simulink model "Simulation"  (R2019b)
settings: Solver=VariableStepAuto  StartTime=0.0  StopTime=tmax  RelTol=1e-3
values from neighbouring files (symbols this model uses):
  BPden = [1 alpha]    [RunSimulation.m]    (also in RunTest.m)
  BPnum = [0.3 alpha]    [RunSimulation.m]    (also in RunTest.m)
  c = 250    [RunSimulation.m]    (also in RunTest.m)
  efficiency = 0.95    [RunSimulation.m]
  Fb = -1*m    (= -90000)    [RunSimulation.m]
  l = 18    [RunSimulation.m]    (also in RunTest.m)
  m = 90000    [RunSimulation.m]
  p0 = 0    [RunSimulation.m]    (also in RunTest.m)
  Pres = 0/1000*[5.7/771 0 1.6]    [RunSimulation.m]    (also in RunTest.m)
  RBD = 5    [RunSimulation.m]    (also in RunTest.m)
  tl = .1    (= 0.1)    [RunSimulation.m]    (also in RunTest.m)
  trackgradient = 0    [RunSimulation.m]    (also in RunTest.m)
  trainpower = m    (= 90000)    [RunSimulation.m]
  v0 = 100/3.6    (= 27.7777777778)    [RunSimulation.m]
  VBD = 3.5    [RunSimulation.m]    (also in RunTest.m)
libraries: simulink x11
(part 1 of 5)
settings Model: Creator=raphael  LastModifiedBy=Westfechtel
settings DataIOCC: ReturnWorkspaceOutputs=off
settings DebuggingCC: ArithmeticOperatorsInVariantConditions=warning
settings SFSimCC: CustomCodeUndefinedFunction=UseInterfaceOnly

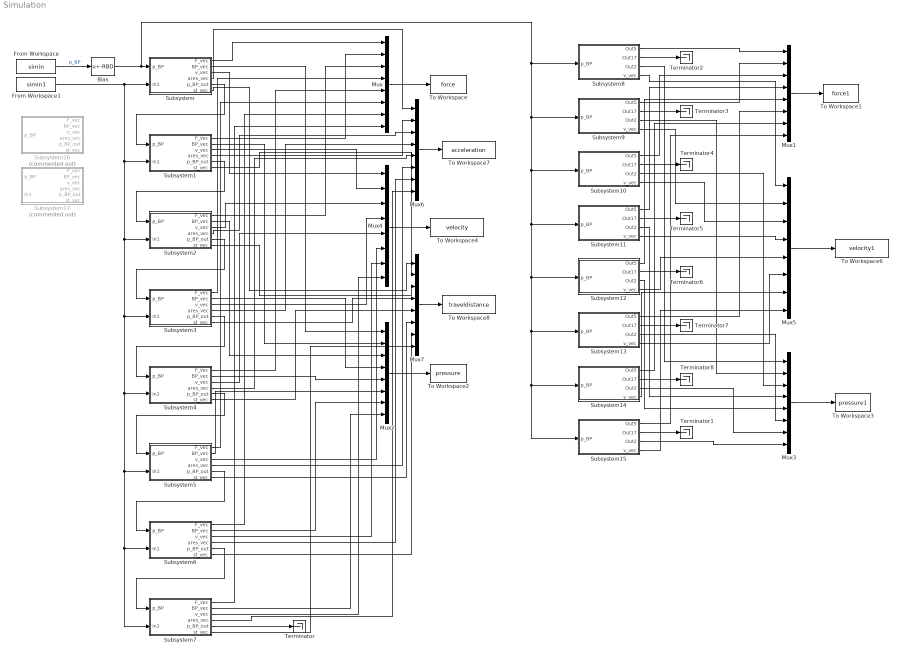
== system Simulation ==
  Bias : Bias  Bias=-RBD
  From Workspace : FromWorkspace  VariableName=simin  SampleTime=0
  From Workspace1 : FromWorkspace  VariableName=simin1  SampleTime=0
  Mux{,1..7} (8 alike) : Mux  Inputs=8
  Subsystem : Subsystem
  Subsystem1 : Subsystem
  Subsystem10 : Subsystem
  Subsystem11 : Subsystem
  Subsystem12 : Subsystem
  Subsystem13 : Subsystem
  Subsystem14 : Subsystem
  Subsystem15 : Subsystem
  Subsystem16 : Subsystem  Commented=on
  Subsystem17 : Subsystem  Commented=on
  Subsystem2 : Subsystem
  Subsystem3 : Subsystem
  Subsystem4 : Subsystem
  Subsystem5 : Subsystem
  Subsystem6 : Subsystem
  Subsystem7 : Subsystem
  Subsystem8 : Subsystem
  Subsystem9 : Subsystem
  Terminator{,1..8} (9 alike) : Terminator
  To Workspace : ToWorkspace  VariableName=force  SaveFormat=Timeseries  SampleTime=-1
  To Workspace1 : ToWorkspace  VariableName=force1  SaveFormat=Timeseries  SampleTime=-1
  To Workspace2 : ToWorkspace  VariableName=pressure  SaveFormat=Timeseries  SampleTime=-1
  To Workspace3 : ToWorkspace  VariableName=pressure1  SaveFormat=Timeseries  SampleTime=-1
  To Workspace4 : ToWorkspace  VariableName=velocity  SaveFormat=Timeseries  SampleTime=-1
  To Workspace6 : ToWorkspace  VariableName=velocity1  SaveFormat=Timeseries  SampleTime=-1
  To Workspace7 : ToWorkspace  VariableName=acceleration  SaveFormat=Timeseries  SampleTime=-1
  To Workspace8 : ToWorkspace  VariableName=traveldistance  SaveFormat=Timeseries  SampleTime=-1
  wires:
  Mux/1 -> To Workspace/1
  Mux2/1 -> To Workspace2/1
  From Workspace/1 -> Bias/1  "p_BP"
  Bias/1 -> Subsystem15/1(p_BP), Subsystem14/1(p_BP), Subsystem13/1(p_BP), Subsystem12/1(p_BP), Subsystem11/1(p_BP), Subsystem10/1(p_BP), Subsystem9/1(p_BP), Subsystem8/1(p_BP), Subsystem/1(p_BP)
  Mux1/1 -> To Workspace1/1
  Mux3/1 -> To Workspace3/1
  Mux4/1 -> To Workspace4/1
  Mux5/1 -> To Workspace6/1
  Subsystem8/2(Out17) -> Terminator2/1
  Subsystem9/2(Out17) -> Terminator3/1
  Subsystem10/2(Out17) -> Terminator4/1
  Subsystem11/2(Out17) -> Terminator5/1
  Subsystem12/2(Out17) -> Terminator6/1
  Subsystem13/2(Out17) -> Terminator7/1
  Subsystem14/2(Out17) -> Terminator8/1
  Subsystem15/2(Out17) -> Terminator1/1
  Subsystem/1(F_vec) -> Mux/1
  Subsystem8/1(Out5) -> Mux1/1
  Subsystem9/1(Out5) -> Mux1/2
  Subsystem10/1(Out5) -> Mux1/3
  Subsystem11/1(Out5) -> Mux1/4
  Subsystem12/1(Out5) -> Mux1/5
  Subsystem13/1(Out5) -> Mux1/6
  Subsystem14/1(Out5) -> Mux1/7
  Subsystem15/1(Out5) -> Mux1/8
  Subsystem8/3(Out2) -> Mux3/1
  Subsystem9/3(Out2) -> Mux3/2
  Subsystem10/3(Out2) -> Mux3/3
  Subsystem11/3(Out2) -> Mux3/4
  Subsystem12/3(Out2) -> Mux3/5
  Subsystem13/3(Out2) -> Mux3/6
  Subsystem14/3(Out2) -> Mux3/7
  Subsystem15/3(Out2) -> Mux3/8
  Subsystem8/4("v_vec ") -> Mux5/1
  Subsystem9/4("v_vec ") -> Mux5/2
  Subsystem10/4("v_vec ") -> Mux5/3
  Subsystem11/4("v_vec ") -> Mux5/4
  Subsystem12/4("v_vec ") -> Mux5/5
  Subsystem13/4("v_vec ") -> Mux5/6
  Subsystem14/4("v_vec ") -> Mux5/7
  Subsystem15/4("v_vec ") -> Mux5/8
  Subsystem7/5(p_BP_out) -> Terminator/1
  Subsystem/5(p_BP_out) -> Subsystem1/1(p_BP)
  Subsystem1/5(p_BP_out) -> Subsystem2/1(p_BP)
  Subsystem2/5(p_BP_out) -> Subsystem3/1(p_BP)
  Subsystem3/5(p_BP_out) -> Subsystem4/1(p_BP)
  Subsystem4/5(p_BP_out) -> Subsystem5/1(p_BP)
  Subsystem5/5(p_BP_out) -> Subsystem6/1(p_BP)
  Subsystem6/5(p_BP_out) -> Subsystem7/1(p_BP)
  Subsystem/2(BP_vec) -> Mux2/1
  Subsystem1/2(BP_vec) -> Mux2/2
  Subsystem1/1(F_vec) -> Mux/2
  Subsystem2/1(F_vec) -> Mux/3
  Subsystem3/1(F_vec) -> Mux/4
  Subsystem4/1(F_vec) -> Mux/5
  Subsystem5/1(F_vec) -> Mux/6
  Subsystem6/1(F_vec) -> Mux/7
  Subsystem7/1(F_vec) -> Mux/8
  Subsystem2/2(BP_vec) -> Mux2/3
  Subsystem3/2(BP_vec) -> Mux2/4
  Subsystem4/2(BP_vec) -> Mux2/5
  Subsystem5/2(BP_vec) -> Mux2/6
  Subsystem6/2(BP_vec) -> Mux2/7
  Subsystem7/2(BP_vec) -> Mux2/8
  Subsystem/3(v_vec) -> Mux4/1
  Subsystem1/3(v_vec) -> Mux4/2
  Subsystem2/3(v_vec) -> Mux4/3
  Subsystem3/3(v_vec) -> Mux4/4
  Subsystem4/3(v_vec) -> Mux4/5
  Subsystem5/3(v_vec) -> Mux4/6
  Subsystem6/3(v_vec) -> Mux4/7
  Subsystem7/3(v_vec) -> Mux4/8
  Mux6/1 -> To Workspace7/1
  Mux7/1 -> To Workspace8/1
  Subsystem/4(ares_vec) -> Mux6/1
  Subsystem1/4(ares_vec) -> Mux6/2
  Subsystem2/4(ares_vec) -> Mux6/3
  Subsystem3/4(ares_vec) -> Mux6/4
  Subsystem4/4(ares_vec) -> Mux6/5
  Subsystem5/4(ares_vec) -> Mux6/6
  Subsystem6/4(ares_vec) -> Mux6/7
  Subsystem7/4(ares_vec) -> Mux6/8
  Subsystem/6(st_vec) -> Mux7/1
  Subsystem1/6(st_vec) -> Mux7/2
  Subsystem2/6(st_vec) -> Mux7/3
  Subsystem3/6(st_vec) -> Mux7/4
  Subsystem4/6(st_vec) -> Mux7/5
  Subsystem5/6(st_vec) -> Mux7/6
  Subsystem6/6(st_vec) -> Mux7/7
  Subsystem7/6(st_vec) -> Mux7/8
  From Workspace1/1 -> Subsystem/2(In1), Subsystem1/2(In1), Subsystem2/2(In1), Subsystem3/2(In1), Subsystem4/2(In1), Subsystem5/2(In1), Subsystem7/2(In1), Subsystem6/2(In1)

== system Simulation/Subsystem ==
  p_BP : Inport
  In1 : Inport  Port=2
  Mux{,1..4} (5 alike) : Mux  Inputs=5
  Wagon model : Subsystem
  Wagon model1 : Subsystem
  Wagon model2 : Subsystem
  Wagon model3 : Subsystem
  Wagon model4 : Subsystem
  F_vec : Outport  VectorParamsAs1DForOutWhenUnconnected=off
  BP_vec : Outport  Port=2  VectorParamsAs1DForOutWhenUnconnected=off
  v_vec : Outport  Port=3  VectorParamsAs1DForOutWhenUnconnected=off
  ares_vec : Outport  Port=4  VectorParamsAs1DForOutWhenUnconnected=off
  p_BP_out : Outport  Port=5  VectorParamsAs1DForOutWhenUnconnected=off
  st_vec : Outport  Port=6  VectorParamsAs1DForOutWhenUnconnected=off
  wires:
  Mux/1 -> F_vec/1  "F_vec"
  p_BP/1 -> Wagon model/1(p_BP)
  Mux1/1 -> BP_vec/1  "BP_vec"
  Mux2/1 -> v_vec/1  "v_vec"
  Mux3/1 -> ares_vec/1  "ares_vec"
  Wagon model4/2(p_BP_out) -> Mux1/5, p_BP_out/1  "p_BP_out"
  Wagon model/1(Fres) -> Mux/1
  Wagon model1/1(Fres) -> Mux/2
  Wagon model2/1(Fres) -> Mux/3
  Wagon model3/1(Fres) -> Mux/4
  Wagon model4/1(Fres) -> Mux/5
  Wagon model/2(p_BP_out) -> Wagon model1/1(p_BP), Mux1/1
  Wagon model1/2(p_BP_out) -> Wagon model2/1(p_BP), Mux1/2
  Wagon model2/2(p_BP_out) -> Wagon model3/1(p_BP), Mux1/3
  Wagon model3/2(p_BP_out) -> Wagon model4/1(p_BP), Mux1/4
  Wagon model/3("v ") -> Mux2/1
  Wagon model1/3("v ") -> Mux2/2
  Wagon model2/3("v ") -> Mux2/3
  Wagon model3/3("v ") -> Mux2/4
  Wagon model4/3("v ") -> Mux2/5
  Wagon model/4(ares) -> Mux3/1
  Wagon model1/4(ares) -> Mux3/2
  Wagon model2/4(ares) -> Mux3/3
  Wagon model3/4(ares) -> Mux3/4
  Wagon model4/4(ares) -> Mux3/5
  Mux4/1 -> st_vec/1  "st_vec"
  Wagon model/5(st) -> Mux4/1
  Wagon model1/5(st) -> Mux4/2
  Wagon model2/5(st) -> Mux4/3
  Wagon model3/5(st) -> Mux4/4
  Wagon model4/5(st) -> Mux4/5
  In1/1 -> Wagon model1/2(In1), Wagon model2/2(In1), Wagon model4/2(In1), Wagon model3/2(In1), Wagon model/2(In1)

== system Simulation/Subsystem1 ==
  p_BP : Inport
  In1 : Inport  Port=2
  Mux{,1..4} (5 alike) : Mux  Inputs=5
  Wagon model : Subsystem
  Wagon model1 : Subsystem
  Wagon model2 : Subsystem
  Wagon model3 : Subsystem
  Wagon model4 : Subsystem
  F_vec : Outport  VectorParamsAs1DForOutWhenUnconnected=off
  BP_vec : Outport  Port=2  VectorParamsAs1DForOutWhenUnconnected=off
  v_vec : Outport  Port=3  VectorParamsAs1DForOutWhenUnconnected=off
  ares_vec : Outport  Port=4  VectorParamsAs1DForOutWhenUnconnected=off
  p_BP_out : Outport  Port=5  VectorParamsAs1DForOutWhenUnconnected=off
  st_vec : Outport  Port=6  VectorParamsAs1DForOutWhenUnconnected=off
  wires:
  Mux/1 -> F_vec/1  "F_vec"
  p_BP/1 -> Wagon model/1(p_BP)
  Mux1/1 -> BP_vec/1  "BP_vec"
  Mux2/1 -> v_vec/1  "v_vec"
  Mux3/1 -> ares_vec/1  "ares_vec"
  Wagon model4/2(p_BP_out) -> Mux1/5, p_BP_out/1  "p_BP_out"
  Wagon model/1(Fres) -> Mux/1
  Wagon model1/1(Fres) -> Mux/2
  Wagon model2/1(Fres) -> Mux/3
  Wagon model3/1(Fres) -> Mux/4
  Wagon model4/1(Fres) -> Mux/5
  Wagon model/2(p_BP_out) -> Wagon model1/1(p_BP), Mux1/1
  Wagon model1/2(p_BP_out) -> Wagon model2/1(p_BP), Mux1/2
  Wagon model2/2(p_BP_out) -> Wagon model3/1(p_BP), Mux1/3
  Wagon model3/2(p_BP_out) -> Wagon model4/1(p_BP), Mux1/4
  Wagon model/3("v ") -> Mux2/1
  Wagon model1/3("v ") -> Mux2/2
  Wagon model2/3("v ") -> Mux2/3
  Wagon model3/3("v ") -> Mux2/4
  Wagon model4/3("v ") -> Mux2/5
  Wagon model/4(ares) -> Mux3/1
  Wagon model1/4(ares) -> Mux3/2
  Wagon model2/4(ares) -> Mux3/3
  Wagon model3/4(ares) -> Mux3/4
  Wagon model4/4(ares) -> Mux3/5
  Mux4/1 -> st_vec/1  "st_vec"
  Wagon model/5(st) -> Mux4/1
  Wagon model1/5(st) -> Mux4/2
  Wagon model2/5(st) -> Mux4/3
  Wagon model3/5(st) -> Mux4/4
  Wagon model4/5(st) -> Mux4/5
  In1/1 -> Wagon model1/2(In1), Wagon model2/2(In1), Wagon model4/2(In1), Wagon model3/2(In1), Wagon model/2(In1)

== system Simulation/Subsystem10 ==
  note: v_vec
  p_BP : Inport
  Mux : Mux  Inputs=5
  Mux1 : Mux  Inputs=5
  Mux2 : Mux  Inputs=5
  Wagon model : Subsystem
  Wagon model1 : Subsystem
  Wagon model2 : Subsystem
  Wagon model3 : Subsystem
  Wagon model4 : Subsystem
  Out5 : Outport  VectorParamsAs1DForOutWhenUnconnected=off
  Out17 : Outport  Port=2  VectorParamsAs1DForOutWhenUnconnected=off
  Out2 : Outport  Port=3  VectorParamsAs1DForOutWhenUnconnected=off
  "v_vec " : Outport  Port=4
  wires:
  Wagon model3/2(p_BP_out) -> Mux2/4, Wagon model4/1(p_BP)
  Mux/1 -> Out5/1  "F_vec"
  Wagon model1/2(p_BP_out) -> Mux2/2, Wagon model2/1(p_BP)
  Wagon model4/2(p_BP_out) -> Out17/1, Mux2/5  "p_BP_out"
  Wagon model4/1(Fres) -> Mux/5
  Wagon model2/2(p_BP_out) -> Mux2/3, Wagon model3/1(p_BP)
  Wagon model/2(p_BP_out) -> Mux2/1, Wagon model1/1(p_BP)
  Wagon model3/1(Fres) -> Mux/4
  Wagon model2/1(Fres) -> Mux/3
  Wagon model1/1(Fres) -> Mux/2
  Wagon model/1(Fres) -> Mux/1
  Mux2/1 -> Out2/1  "BP_vec"
  p_BP/1 -> Wagon model/1(p_BP)
  Wagon model/3("v ") -> Mux1/1
  Wagon model1/3("v ") -> Mux1/2
  Wagon model3/3("v ") -> Mux1/3
  Wagon model4/3("v ") -> Mux1/5
  Wagon model2/3("v ") -> Mux1/4
  Mux1/1 -> "v_vec "/1

== system Simulation/Subsystem11 ==
  note: v_vec
  p_BP : Inport
  Mux : Mux  Inputs=5
  Mux1 : Mux  Inputs=5
  Mux2 : Mux  Inputs=5
  Wagon model : Subsystem
  Wagon model1 : Subsystem
  Wagon model2 : Subsystem
  Wagon model3 : Subsystem
  Wagon model4 : Subsystem
  Out5 : Outport  VectorParamsAs1DForOutWhenUnconnected=off
  Out17 : Outport  Port=2  VectorParamsAs1DForOutWhenUnconnected=off
  Out2 : Outport  Port=3  VectorParamsAs1DForOutWhenUnconnected=off
  "v_vec " : Outport  Port=4
  wires:
  Wagon model3/2(p_BP_out) -> Mux2/4, Wagon model4/1(p_BP)
  Mux/1 -> Out5/1  "F_vec"
  Wagon model1/2(p_BP_out) -> Mux2/2, Wagon model2/1(p_BP)
  Wagon model4/2(p_BP_out) -> Out17/1, Mux2/5  "p_BP_out"
  Wagon model4/1(Fres) -> Mux/5
  Wagon model2/2(p_BP_out) -> Mux2/3, Wagon model3/1(p_BP)
  Wagon model/2(p_BP_out) -> Mux2/1, Wagon model1/1(p_BP)
  Wagon model3/1(Fres) -> Mux/4
  Wagon model2/1(Fres) -> Mux/3
  Wagon model1/1(Fres) -> Mux/2
  Wagon model/1(Fres) -> Mux/1
  Mux2/1 -> Out2/1  "BP_vec"
  p_BP/1 -> Wagon model/1(p_BP)
  Wagon model/3("v ") -> Mux1/1
  Wagon model1/3("v ") -> Mux1/2
  Wagon model3/3("v ") -> Mux1/3
  Wagon model4/3("v ") -> Mux1/5
  Wagon model2/3("v ") -> Mux1/4
  Mux1/1 -> "v_vec "/1

== system Simulation/Subsystem12 ==
  note: v_vec
  p_BP : Inport
  Mux : Mux  Inputs=5
  Mux1 : Mux  Inputs=5
  Mux2 : Mux  Inputs=5
  Wagon model : Subsystem
  Wagon model1 : Subsystem
  Wagon model2 : Subsystem
  Wagon model3 : Subsystem
  Wagon model4 : Subsystem
  Out5 : Outport  VectorParamsAs1DForOutWhenUnconnected=off
  Out17 : Outport  Port=2  VectorParamsAs1DForOutWhenUnconnected=off
  Out2 : Outport  Port=3  VectorParamsAs1DForOutWhenUnconnected=off
  "v_vec " : Outport  Port=4
  wires:
  Wagon model3/2(p_BP_out) -> Mux2/4, Wagon model4/1(p_BP)
  Mux/1 -> Out5/1  "F_vec"
  Wagon model1/2(p_BP_out) -> Mux2/2, Wagon model2/1(p_BP)
  Wagon model4/2(p_BP_out) -> Out17/1, Mux2/5  "p_BP_out"
  Wagon model4/1(Fres) -> Mux/5
  Wagon model2/2(p_BP_out) -> Mux2/3, Wagon model3/1(p_BP)
  Wagon model/2(p_BP_out) -> Mux2/1, Wagon model1/1(p_BP)
  Wagon model3/1(Fres) -> Mux/4
  Wagon model2/1(Fres) -> Mux/3
  Wagon model1/1(Fres) -> Mux/2
  Wagon model/1(Fres) -> Mux/1
  Mux2/1 -> Out2/1  "BP_vec"
  p_BP/1 -> Wagon model/1(p_BP)
  Wagon model/3("v ") -> Mux1/1
  Wagon model1/3("v ") -> Mux1/2
  Wagon model3/3("v ") -> Mux1/3
  Wagon model4/3("v ") -> Mux1/5
  Wagon model2/3("v ") -> Mux1/4
  Mux1/1 -> "v_vec "/1

== system Simulation/Subsystem13 ==
  note: v_vec
  p_BP : Inport
  Mux : Mux  Inputs=5
  Mux1 : Mux  Inputs=5
  Mux2 : Mux  Inputs=5
  Wagon model : Subsystem
  Wagon model1 : Subsystem
  Wagon model2 : Subsystem
  Wagon model3 : Subsystem
  Wagon model4 : Subsystem
  Out5 : Outport  VectorParamsAs1DForOutWhenUnconnected=off
  Out17 : Outport  Port=2  VectorParamsAs1DForOutWhenUnconnected=off
  Out2 : Outport  Port=3  VectorParamsAs1DForOutWhenUnconnected=off
  "v_vec " : Outport  Port=4
  wires:
  Wagon model3/2(p_BP_out) -> Mux2/4, Wagon model4/1(p_BP)
  Mux/1 -> Out5/1  "F_vec"
  Wagon model1/2(p_BP_out) -> Mux2/2, Wagon model2/1(p_BP)
  Wagon model4/2(p_BP_out) -> Out17/1, Mux2/5  "p_BP_out"
  Wagon model4/1(Fres) -> Mux/5
  Wagon model2/2(p_BP_out) -> Mux2/3, Wagon model3/1(p_BP)
  Wagon model/2(p_BP_out) -> Mux2/1, Wagon model1/1(p_BP)
  Wagon model3/1(Fres) -> Mux/4
  Wagon model2/1(Fres) -> Mux/3
  Wagon model1/1(Fres) -> Mux/2
  Wagon model/1(Fres) -> Mux/1
  Mux2/1 -> Out2/1  "BP_vec"
  p_BP/1 -> Wagon model/1(p_BP)
  Wagon model/3("v ") -> Mux1/1
  Wagon model1/3("v ") -> Mux1/2
  Wagon model3/3("v ") -> Mux1/3
  Wagon model4/3("v ") -> Mux1/5
  Wagon model2/3("v ") -> Mux1/4
  Mux1/1 -> "v_vec "/1

== system Simulation/Subsystem14 ==
  note: v_vec
  p_BP : Inport
  Mux : Mux  Inputs=5
  Mux1 : Mux  Inputs=5
  Mux2 : Mux  Inputs=5
  Wagon model : Subsystem
  Wagon model1 : Subsystem
  Wagon model2 : Subsystem
  Wagon model3 : Subsystem
  Wagon model4 : Subsystem
  Out5 : Outport  VectorParamsAs1DForOutWhenUnconnected=off
  Out17 : Outport  Port=2  VectorParamsAs1DForOutWhenUnconnected=off
  Out2 : Outport  Port=3  VectorParamsAs1DForOutWhenUnconnected=off
  "v_vec " : Outport  Port=4
  wires:
  Wagon model3/2(p_BP_out) -> Mux2/4, Wagon model4/1(p_BP)
  Mux/1 -> Out5/1  "F_vec"
  Wagon model1/2(p_BP_out) -> Mux2/2, Wagon model2/1(p_BP)
  Wagon model4/2(p_BP_out) -> Out17/1, Mux2/5  "p_BP_out"
  Wagon model4/1(Fres) -> Mux/5
  Wagon model2/2(p_BP_out) -> Mux2/3, Wagon model3/1(p_BP)
  Wagon model/2(p_BP_out) -> Mux2/1, Wagon model1/1(p_BP)
  Wagon model3/1(Fres) -> Mux/4
  Wagon model2/1(Fres) -> Mux/3
  Wagon model1/1(Fres) -> Mux/2
  Wagon model/1(Fres) -> Mux/1
  Mux2/1 -> Out2/1  "BP_vec"
  p_BP/1 -> Wagon model/1(p_BP)
  Wagon model/3("v ") -> Mux1/1
  Wagon model1/3("v ") -> Mux1/2
  Wagon model3/3("v ") -> Mux1/3
  Wagon model4/3("v ") -> Mux1/5
  Wagon model2/3("v ") -> Mux1/4
  Mux1/1 -> "v_vec "/1

== system Simulation/Subsystem15 ==
  note: v_vec
  p_BP : Inport
  Mux : Mux  Inputs=5
  Mux1 : Mux  Inputs=5
  Mux2 : Mux  Inputs=5
  Wagon model : Subsystem
  Wagon model1 : Subsystem
  Wagon model2 : Subsystem
  Wagon model3 : Subsystem
  Wagon model4 : Subsystem
  Out5 : Outport  VectorParamsAs1DForOutWhenUnconnected=off
  Out17 : Outport  Port=2  VectorParamsAs1DForOutWhenUnconnected=off
  Out2 : Outport  Port=3  VectorParamsAs1DForOutWhenUnconnected=off
  "v_vec " : Outport  Port=4
  wires:
  Wagon model3/2(p_BP_out) -> Mux2/4, Wagon model4/1(p_BP)
  Mux/1 -> Out5/1  "F_vec"
  Wagon model1/2(p_BP_out) -> Mux2/2, Wagon model2/1(p_BP)
  Wagon model4/2(p_BP_out) -> Out17/1, Mux2/5  "p_BP_out"
  Wagon model4/1(Fres) -> Mux/5
  Wagon model2/2(p_BP_out) -> Mux2/3, Wagon model3/1(p_BP)
  Wagon model/2(p_BP_out) -> Mux2/1, Wagon model1/1(p_BP)
  Wagon model3/1(Fres) -> Mux/4
  Wagon model2/1(Fres) -> Mux/3
  Wagon model1/1(Fres) -> Mux/2
  Wagon model/1(Fres) -> Mux/1
  Mux2/1 -> Out2/1  "BP_vec"
  p_BP/1 -> Wagon model/1(p_BP)
  Wagon model/3("v ") -> Mux1/1
  Wagon model1/3("v ") -> Mux1/2
  Wagon model3/3("v ") -> Mux1/3
  Wagon model4/3("v ") -> Mux1/5
  Wagon model2/3("v ") -> Mux1/4
  Mux1/1 -> "v_vec "/1

== system Simulation/Subsystem16 ==
  p_BP : Inport
  Mux{,1..4} (5 alike) : Mux  Inputs=5
  Wagon model : Subsystem
  Wagon model1 : Subsystem
  Wagon model2 : Subsystem
  Wagon model3 : Subsystem
  Wagon model4 : Subsystem
  F_vec : Outport  VectorParamsAs1DForOutWhenUnconnected=off
  BP_vec : Outport  Port=2  VectorParamsAs1DForOutWhenUnconnected=off
  v_vec : Outport  Port=3  VectorParamsAs1DForOutWhenUnconnected=off
  ares_vec : Outport  Port=4  VectorParamsAs1DForOutWhenUnconnected=off
  p_BP_out : Outport  Port=5  VectorParamsAs1DForOutWhenUnconnected=off
  st_vec : Outport  Port=6  VectorParamsAs1DForOutWhenUnconnected=off
  wires:
  Mux/1 -> F_vec/1  "F_vec"
  p_BP/1 -> Wagon model/1(p_BP)
  Mux1/1 -> BP_vec/1  "BP_vec"
  Mux2/1 -> v_vec/1  "v_vec"
  Mux3/1 -> ares_vec/1  "ares_vec"
  Wagon model4/2(p_BP_out) -> Mux1/5, p_BP_out/1  "p_BP_out"
  Wagon model/1(Fres) -> Mux/1
  Wagon model1/1(Fres) -> Mux/2
  Wagon model2/1(Fres) -> Mux/3
  Wagon model3/1(Fres) -> Mux/4
  Wagon model4/1(Fres) -> Mux/5
  Wagon model/2(p_BP_out) -> Wagon model1/1(p_BP), Mux1/1
  Wagon model1/2(p_BP_out) -> Wagon model2/1(p_BP), Mux1/2
  Wagon model2/2(p_BP_out) -> Wagon model3/1(p_BP), Mux1/3
  Wagon model3/2(p_BP_out) -> Wagon model4/1(p_BP), Mux1/4
  Wagon model/3("v ") -> Mux2/1
  Wagon model1/3("v ") -> Mux2/2
  Wagon model2/3("v ") -> Mux2/3
  Wagon model3/3("v ") -> Mux2/4
  Wagon model4/3("v ") -> Mux2/5
  Wagon model/4(ares) -> Mux3/1
  Wagon model1/4(ares) -> Mux3/2
  Wagon model2/4(ares) -> Mux3/3
  Wagon model3/4(ares) -> Mux3/4
  Wagon model4/4(ares) -> Mux3/5
  Mux4/1 -> st_vec/1  "st_vec"
  Wagon model/5(st) -> Mux4/1
  Wagon model1/5(st) -> Mux4/2
  Wagon model2/5(st) -> Mux4/3
  Wagon model3/5(st) -> Mux4/4
  Wagon model4/5(st) -> Mux4/5

== system Simulation/Subsystem17 ==
  p_BP : Inport
  In1 : Inport  Port=2
  Mux{,1..4} (5 alike) : Mux  Inputs=5
  Wagon model : Subsystem
  Wagon model1 : Subsystem
  Wagon model2 : Subsystem
  Wagon model3 : Subsystem
  Wagon model4 : Subsystem
  F_vec : Outport  VectorParamsAs1DForOutWhenUnconnected=off
  BP_vec : Outport  Port=2  VectorParamsAs1DForOutWhenUnconnected=off
  v_vec : Outport  Port=3  VectorParamsAs1DForOutWhenUnconnected=off
  ares_vec : Outport  Port=4  VectorParamsAs1DForOutWhenUnconnected=off
  p_BP_out : Outport  Port=5  VectorParamsAs1DForOutWhenUnconnected=off
  st_vec : Outport  Port=6  VectorParamsAs1DForOutWhenUnconnected=off
  wires:
  Mux/1 -> F_vec/1  "F_vec"
  p_BP/1 -> Wagon model/1(p_BP)
  Mux1/1 -> BP_vec/1  "BP_vec"
  Mux2/1 -> v_vec/1  "v_vec"
  Mux3/1 -> ares_vec/1  "ares_vec"
  Wagon model4/2(p_BP_out) -> Mux1/5, p_BP_out/1  "p_BP_out"
  Wagon model/1(Fres) -> Mux/1
  Wagon model1/1(Fres) -> Mux/2
  Wagon model2/1(Fres) -> Mux/3
  Wagon model3/1(Fres) -> Mux/4
  Wagon model4/1(Fres) -> Mux/5
  Wagon model/2(p_BP_out) -> Wagon model1/1(p_BP), Mux1/1
  Wagon model1/2(p_BP_out) -> Wagon model2/1(p_BP), Mux1/2
  Wagon model2/2(p_BP_out) -> Wagon model3/1(p_BP), Mux1/3
  Wagon model3/2(p_BP_out) -> Wagon model4/1(p_BP), Mux1/4
  Wagon model/3("v ") -> Mux2/1
  Wagon model1/3("v ") -> Mux2/2
  Wagon model2/3("v ") -> Mux2/3
  Wagon model3/3("v ") -> Mux2/4
  Wagon model4/3("v ") -> Mux2/5
  Wagon model/4(ares) -> Mux3/1
  Wagon model1/4(ares) -> Mux3/2
  Wagon model2/4(ares) -> Mux3/3
  Wagon model3/4(ares) -> Mux3/4
  Wagon model4/4(ares) -> Mux3/5
  Mux4/1 -> st_vec/1  "st_vec"
  Wagon model/5(st) -> Mux4/1
  Wagon model1/5(st) -> Mux4/2
  Wagon model2/5(st) -> Mux4/3
  Wagon model3/5(st) -> Mux4/4
  Wagon model4/5(st) -> Mux4/5
  In1/1 -> Wagon model4/2(In1), Wagon model3/2(In1), Wagon model2/2(In1), Wagon model1/2(In1), Wagon model/2(In1)

== system Simulation/Subsystem2 ==
  p_BP : Inport
  In1 : Inport  Port=2
  Mux{,1..4} (5 alike) : Mux  Inputs=5
  Wagon model : Subsystem
  Wagon model1 : Subsystem
  Wagon model2 : Subsystem
  Wagon model3 : Subsystem
  Wagon model4 : Subsystem
  F_vec : Outport  VectorParamsAs1DForOutWhenUnconnected=off
  BP_vec : Outport  Port=2  VectorParamsAs1DForOutWhenUnconnected=off
  v_vec : Outport  Port=3  VectorParamsAs1DForOutWhenUnconnected=off
  ares_vec : Outport  Port=4  VectorParamsAs1DForOutWhenUnconnected=off
  p_BP_out : Outport  Port=5  VectorParamsAs1DForOutWhenUnconnected=off
  st_vec : Outport  Port=6  VectorParamsAs1DForOutWhenUnconnected=off
  wires:
  Mux/1 -> F_vec/1  "F_vec"
  p_BP/1 -> Wagon model/1(p_BP)
  Mux1/1 -> BP_vec/1  "BP_vec"
  Mux2/1 -> v_vec/1  "v_vec"
  Mux3/1 -> ares_vec/1  "ares_vec"
  Wagon model4/2(p_BP_out) -> Mux1/5, p_BP_out/1  "p_BP_out"
  Wagon model/1(Fres) -> Mux/1
  Wagon model1/1(Fres) -> Mux/2
  Wagon model2/1(Fres) -> Mux/3
  Wagon model3/1(Fres) -> Mux/4
  Wagon model4/1(Fres) -> Mux/5
  Wagon model/2(p_BP_out) -> Wagon model1/1(p_BP), Mux1/1
  Wagon model1/2(p_BP_out) -> Wagon model2/1(p_BP), Mux1/2
  Wagon model2/2(p_BP_out) -> Wagon model3/1(p_BP), Mux1/3
  Wagon model3/2(p_BP_out) -> Wagon model4/1(p_BP), Mux1/4
  Wagon model/3("v ") -> Mux2/1
  Wagon model1/3("v ") -> Mux2/2
  Wagon model2/3("v ") -> Mux2/3
  Wagon model3/3("v ") -> Mux2/4
  Wagon model4/3("v ") -> Mux2/5
  Wagon model/4(ares) -> Mux3/1
  Wagon model1/4(ares) -> Mux3/2
  Wagon model2/4(ares) -> Mux3/3
  Wagon model3/4(ares) -> Mux3/4
  Wagon model4/4(ares) -> Mux3/5
  Mux4/1 -> st_vec/1  "st_vec"
  Wagon model/5(st) -> Mux4/1
  Wagon model1/5(st) -> Mux4/2
  Wagon model2/5(st) -> Mux4/3
  Wagon model3/5(st) -> Mux4/4
  Wagon model4/5(st) -> Mux4/5
  In1/1 -> Wagon model1/2(In1), Wagon model2/2(In1), Wagon model4/2(In1), Wagon model3/2(In1), Wagon model/2(In1)

== system Simulation/Subsystem3 ==
  p_BP : Inport
  In1 : Inport  Port=2
  Mux{,1..4} (5 alike) : Mux  Inputs=5
  Wagon model : Subsystem
  Wagon model1 : Subsystem
  Wagon model2 : Subsystem
  Wagon model3 : Subsystem
  Wagon model4 : Subsystem
  F_vec : Outport  VectorParamsAs1DForOutWhenUnconnected=off
  BP_vec : Outport  Port=2  VectorParamsAs1DForOutWhenUnconnected=off
  v_vec : Outport  Port=3  VectorParamsAs1DForOutWhenUnconnected=off
  ares_vec : Outport  Port=4  VectorParamsAs1DForOutWhenUnconnected=off
  p_BP_out : Outport  Port=5  VectorParamsAs1DForOutWhenUnconnected=off
  st_vec : Outport  Port=6  VectorParamsAs1DForOutWhenUnconnected=off
  wires:
  Mux/1 -> F_vec/1  "F_vec"
  p_BP/1 -> Wagon model/1(p_BP)
  Mux1/1 -> BP_vec/1  "BP_vec"
  Mux2/1 -> v_vec/1  "v_vec"
  Mux3/1 -> ares_vec/1  "ares_vec"
  Wagon model4/2(p_BP_out) -> Mux1/5, p_BP_out/1  "p_BP_out"
  Wagon model/1(Fres) -> Mux/1
  Wagon model1/1(Fres) -> Mux/2
  Wagon model2/1(Fres) -> Mux/3
  Wagon model3/1(Fres) -> Mux/4
  Wagon model4/1(Fres) -> Mux/5
  Wagon model/2(p_BP_out) -> Wagon model1/1(p_BP), Mux1/1
  Wagon model1/2(p_BP_out) -> Wagon model2/1(p_BP), Mux1/2
  Wagon model2/2(p_BP_out) -> Wagon model3/1(p_BP), Mux1/3
  Wagon model3/2(p_BP_out) -> Wagon model4/1(p_BP), Mux1/4
  Wagon model/3("v ") -> Mux2/1
  Wagon model1/3("v ") -> Mux2/2
  Wagon model2/3("v ") -> Mux2/3
  Wagon model3/3("v ") -> Mux2/4
  Wagon model4/3("v ") -> Mux2/5
  Wagon model/4(ares) -> Mux3/1
  Wagon model1/4(ares) -> Mux3/2
  Wagon model2/4(ares) -> Mux3/3
  Wagon model3/4(ares) -> Mux3/4
  Wagon model4/4(ares) -> Mux3/5
  Mux4/1 -> st_vec/1  "st_vec"
  Wagon model/5(st) -> Mux4/1
  Wagon model1/5(st) -> Mux4/2
  Wagon model2/5(st) -> Mux4/3
  Wagon model3/5(st) -> Mux4/4
  Wagon model4/5(st) -> Mux4/5
  In1/1 -> Wagon model1/2(In1), Wagon model2/2(In1), Wagon model4/2(In1), Wagon model3/2(In1), Wagon model/2(In1)

== system Simulation/Subsystem4 ==
  p_BP : Inport
  In1 : Inport  Port=2
  Mux{,1..4} (5 alike) : Mux  Inputs=5
  Wagon model : Subsystem
  Wagon model1 : Subsystem
  Wagon model2 : Subsystem
  Wagon model3 : Subsystem
  Wagon model4 : Subsystem
  F_vec : Outport  VectorParamsAs1DForOutWhenUnconnected=off
  BP_vec : Outport  Port=2  VectorParamsAs1DForOutWhenUnconnected=off
  v_vec : Outport  Port=3  VectorParamsAs1DForOutWhenUnconnected=off
  ares_vec : Outport  Port=4  VectorParamsAs1DForOutWhenUnconnected=off
  p_BP_out : Outport  Port=5  VectorParamsAs1DForOutWhenUnconnected=off
  st_vec : Outport  Port=6  VectorParamsAs1DForOutWhenUnconnected=off
  wires:
  Mux/1 -> F_vec/1  "F_vec"
  p_BP/1 -> Wagon model/1(p_BP)
  Mux1/1 -> BP_vec/1  "BP_vec"
  Mux2/1 -> v_vec/1  "v_vec"
  Mux3/1 -> ares_vec/1  "ares_vec"
  Wagon model4/2(p_BP_out) -> Mux1/5, p_BP_out/1  "p_BP_out"
  Wagon model/1(Fres) -> Mux/1
  Wagon model1/1(Fres) -> Mux/2
  Wagon model2/1(Fres) -> Mux/3
  Wagon model3/1(Fres) -> Mux/4
  Wagon model4/1(Fres) -> Mux/5
  Wagon model/2(p_BP_out) -> Wagon model1/1(p_BP), Mux1/1
  Wagon model1/2(p_BP_out) -> Wagon model2/1(p_BP), Mux1/2
  Wagon model2/2(p_BP_out) -> Wagon model3/1(p_BP), Mux1/3
  Wagon model3/2(p_BP_out) -> Wagon model4/1(p_BP), Mux1/4
  Wagon model/3("v ") -> Mux2/1
  Wagon model1/3("v ") -> Mux2/2
  Wagon model2/3("v ") -> Mux2/3
  Wagon model3/3("v ") -> Mux2/4
  Wagon model4/3("v ") -> Mux2/5
  Wagon model/4(ares) -> Mux3/1
  Wagon model1/4(ares) -> Mux3/2
  Wagon model2/4(ares) -> Mux3/3
  Wagon model3/4(ares) -> Mux3/4
  Wagon model4/4(ares) -> Mux3/5
  Mux4/1 -> st_vec/1  "st_vec"
  Wagon model/5(st) -> Mux4/1
  Wagon model1/5(st) -> Mux4/2
  Wagon model2/5(st) -> Mux4/3
  Wagon model3/5(st) -> Mux4/4
  Wagon model4/5(st) -> Mux4/5
  In1/1 -> Wagon model1/2(In1), Wagon model2/2(In1), Wagon model4/2(In1), Wagon model3/2(In1), Wagon model/2(In1)

== system Simulation/Subsystem5 ==
  p_BP : Inport
  In1 : Inport  Port=2
  Mux{,1..4} (5 alike) : Mux  Inputs=5
  Wagon model : Subsystem
  Wagon model1 : Subsystem
  Wagon model2 : Subsystem
  Wagon model3 : Subsystem
  Wagon model4 : Subsystem
  F_vec : Outport  VectorParamsAs1DForOutWhenUnconnected=off
  BP_vec : Outport  Port=2  VectorParamsAs1DForOutWhenUnconnected=off
  v_vec : Outport  Port=3  VectorParamsAs1DForOutWhenUnconnected=off
  ares_vec : Outport  Port=4  VectorParamsAs1DForOutWhenUnconnected=off
  p_BP_out : Outport  Port=5  VectorParamsAs1DForOutWhenUnconnected=off
  st_vec : Outport  Port=6  VectorParamsAs1DForOutWhenUnconnected=off
  wires:
  Mux/1 -> F_vec/1  "F_vec"
  p_BP/1 -> Wagon model/1(p_BP)
  Mux1/1 -> BP_vec/1  "BP_vec"
  Mux2/1 -> v_vec/1  "v_vec"
  Mux3/1 -> ares_vec/1  "ares_vec"
  Wagon model4/2(p_BP_out) -> Mux1/5, p_BP_out/1  "p_BP_out"
  Wagon model/1(Fres) -> Mux/1
  Wagon model1/1(Fres) -> Mux/2
  Wagon model2/1(Fres) -> Mux/3
  Wagon model3/1(Fres) -> Mux/4
  Wagon model4/1(Fres) -> Mux/5
  Wagon model/2(p_BP_out) -> Wagon model1/1(p_BP), Mux1/1
  Wagon model1/2(p_BP_out) -> Wagon model2/1(p_BP), Mux1/2
  Wagon model2/2(p_BP_out) -> Wagon model3/1(p_BP), Mux1/3
  Wagon model3/2(p_BP_out) -> Wagon model4/1(p_BP), Mux1/4
  Wagon model/3("v ") -> Mux2/1
  Wagon model1/3("v ") -> Mux2/2
  Wagon model2/3("v ") -> Mux2/3
  Wagon model3/3("v ") -> Mux2/4
  Wagon model4/3("v ") -> Mux2/5
  Wagon model/4(ares) -> Mux3/1
  Wagon model1/4(ares) -> Mux3/2
  Wagon model2/4(ares) -> Mux3/3
  Wagon model3/4(ares) -> Mux3/4
  Wagon model4/4(ares) -> Mux3/5
  Mux4/1 -> st_vec/1  "st_vec"
  Wagon model/5(st) -> Mux4/1
  Wagon model1/5(st) -> Mux4/2
  Wagon model2/5(st) -> Mux4/3
  Wagon model3/5(st) -> Mux4/4
  Wagon model4/5(st) -> Mux4/5
  In1/1 -> Wagon model1/2(In1), Wagon model2/2(In1), Wagon model4/2(In1), Wagon model3/2(In1), Wagon model/2(In1)

== system Simulation/Subsystem6 ==
  p_BP : Inport
  In1 : Inport  Port=2
  Mux{,1..4} (5 alike) : Mux  Inputs=5
  Wagon model : Subsystem
  Wagon model1 : Subsystem
  Wagon model2 : Subsystem
  Wagon model3 : Subsystem
  Wagon model4 : Subsystem
  F_vec : Outport  VectorParamsAs1DForOutWhenUnconnected=off
  BP_vec : Outport  Port=2  VectorParamsAs1DForOutWhenUnconnected=off
  v_vec : Outport  Port=3  VectorParamsAs1DForOutWhenUnconnected=off
  ares_vec : Outport  Port=4  VectorParamsAs1DForOutWhenUnconnected=off
  p_BP_out : Outport  Port=5  VectorParamsAs1DForOutWhenUnconnected=off
  st_vec : Outport  Port=6  VectorParamsAs1DForOutWhenUnconnected=off
  wires:
  Mux/1 -> F_vec/1  "F_vec"
  p_BP/1 -> Wagon model/1(p_BP)
  Mux1/1 -> BP_vec/1  "BP_vec"
  Mux2/1 -> v_vec/1  "v_vec"
  Mux3/1 -> ares_vec/1  "ares_vec"
  Wagon model4/2(p_BP_out) -> Mux1/5, p_BP_out/1  "p_BP_out"
  Wagon model/1(Fres) -> Mux/1
  Wagon model1/1(Fres) -> Mux/2
  Wagon model2/1(Fres) -> Mux/3
  Wagon model3/1(Fres) -> Mux/4
  Wagon model4/1(Fres) -> Mux/5
  Wagon model/2(p_BP_out) -> Wagon model1/1(p_BP), Mux1/1
  Wagon model1/2(p_BP_out) -> Wagon model2/1(p_BP), Mux1/2
  Wagon model2/2(p_BP_out) -> Wagon model3/1(p_BP), Mux1/3
  Wagon model3/2(p_BP_out) -> Wagon model4/1(p_BP), Mux1/4
  Wagon model/3("v ") -> Mux2/1
  Wagon model1/3("v ") -> Mux2/2
  Wagon model2/3("v ") -> Mux2/3
  Wagon model3/3("v ") -> Mux2/4
  Wagon model4/3("v ") -> Mux2/5
  Wagon model/4(ares) -> Mux3/1
  Wagon model1/4(ares) -> Mux3/2
  Wagon model2/4(ares) -> Mux3/3
  Wagon model3/4(ares) -> Mux3/4
  Wagon model4/4(ares) -> Mux3/5
  Mux4/1 -> st_vec/1  "st_vec"
  Wagon model/5(st) -> Mux4/1
  Wagon model1/5(st) -> Mux4/2
  Wagon model2/5(st) -> Mux4/3
  Wagon model3/5(st) -> Mux4/4
  Wagon model4/5(st) -> Mux4/5
  In1/1 -> Wagon model1/2(In1), Wagon model2/2(In1), Wagon model4/2(In1), Wagon model3/2(In1), Wagon model/2(In1)

== system Simulation/Subsystem7 ==
  p_BP : Inport
  In1 : Inport  Port=2
  Mux{,1..4} (5 alike) : Mux  Inputs=5
  Wagon model : Subsystem
  Wagon model1 : Subsystem
  Wagon model2 : Subsystem
  Wagon model3 : Subsystem
  Wagon model4 : Subsystem
  F_vec : Outport  VectorParamsAs1DForOutWhenUnconnected=off
  BP_vec : Outport  Port=2  VectorParamsAs1DForOutWhenUnconnected=off
  v_vec : Outport  Port=3  VectorParamsAs1DForOutWhenUnconnected=off
  ares_vec : Outport  Port=4  VectorParamsAs1DForOutWhenUnconnected=off
  p_BP_out : Outport  Port=5  VectorParamsAs1DForOutWhenUnconnected=off
  st_vec : Outport  Port=6  VectorParamsAs1DForOutWhenUnconnected=off
  wires:
  Mux/1 -> F_vec/1  "F_vec"
  p_BP/1 -> Wagon model/1(p_BP)
  Mux1/1 -> BP_vec/1  "BP_vec"
  Mux2/1 -> v_vec/1  "v_vec"
  Mux3/1 -> ares_vec/1  "ares_vec"
  Wagon model4/2(p_BP_out) -> Mux1/5, p_BP_out/1  "p_BP_out"
  Wagon model/1(Fres) -> Mux/1
  Wagon model1/1(Fres) -> Mux/2
  Wagon model2/1(Fres) -> Mux/3
  Wagon model3/1(Fres) -> Mux/4
  Wagon model4/1(Fres) -> Mux/5
  Wagon model/2(p_BP_out) -> Wagon model1/1(p_BP), Mux1/1
  Wagon model1/2(p_BP_out) -> Wagon model2/1(p_BP), Mux1/2
  Wagon model2/2(p_BP_out) -> Wagon model3/1(p_BP), Mux1/3
  Wagon model3/2(p_BP_out) -> Wagon model4/1(p_BP), Mux1/4
  Wagon model/3("v ") -> Mux2/1
  Wagon model1/3("v ") -> Mux2/2
  Wagon model2/3("v ") -> Mux2/3
  Wagon model3/3("v ") -> Mux2/4
  Wagon model4/3("v ") -> Mux2/5
  Wagon model/4(ares) -> Mux3/1
  Wagon model1/4(ares) -> Mux3/2
  Wagon model2/4(ares) -> Mux3/3
  Wagon model3/4(ares) -> Mux3/4
  Wagon model4/4(ares) -> Mux3/5
  Mux4/1 -> st_vec/1  "st_vec"
  Wagon model/5(st) -> Mux4/1
  Wagon model1/5(st) -> Mux4/2
  Wagon model2/5(st) -> Mux4/3
  Wagon model3/5(st) -> Mux4/4
  Wagon model4/5(st) -> Mux4/5
  In1/1 -> Wagon model1/2(In1), Wagon model2/2(In1), Wagon model4/2(In1), Wagon model3/2(In1), Wagon model/2(In1)

== system Simulation/Subsystem8 ==
  note: v_vec
  p_BP : Inport
  Mux : Mux  Inputs=5
  Mux1 : Mux  Inputs=5
  Mux2 : Mux  Inputs=5
  Wagon model : Subsystem
  Wagon model1 : Subsystem
  Wagon model2 : Subsystem
  Wagon model3 : Subsystem
  Wagon model4 : Subsystem
  Out5 : Outport  VectorParamsAs1DForOutWhenUnconnected=off
  Out17 : Outport  Port=2  VectorParamsAs1DForOutWhenUnconnected=off
  Out2 : Outport  Port=3  VectorParamsAs1DForOutWhenUnconnected=off
  "v_vec " : Outport  Port=4
  wires:
  Wagon model3/2(p_BP_out) -> Mux2/4, Wagon model4/1(p_BP)
  Mux/1 -> Out5/1  "F_vec"
  Wagon model1/2(p_BP_out) -> Mux2/2, Wagon model2/1(p_BP)
  Wagon model4/2(p_BP_out) -> Out17/1, Mux2/5  "p_BP_out"
  Wagon model4/1(Fres) -> Mux/5
  Wagon model2/2(p_BP_out) -> Mux2/3, Wagon model3/1(p_BP)
  Wagon model/2(p_BP_out) -> Mux2/1, Wagon model1/1(p_BP)
  Wagon model3/1(Fres) -> Mux/4
  Wagon model2/1(Fres) -> Mux/3
  Wagon model1/1(Fres) -> Mux/2
  Wagon model/1(Fres) -> Mux/1
  Mux2/1 -> Out2/1  "BP_vec"
  p_BP/1 -> Wagon model/1(p_BP)
  Wagon model/3("v ") -> Mux1/1
  Wagon model1/3("v ") -> Mux1/2
  Wagon model3/3("v ") -> Mux1/3
  Wagon model4/3("v ") -> Mux1/5
  Wagon model2/3("v ") -> Mux1/4
  Mux1/1 -> "v_vec "/1

== system Simulation/Subsystem9 ==
  note: v_vec
  p_BP : Inport
  Mux : Mux  Inputs=5
  Mux1 : Mux  Inputs=5
  Mux2 : Mux  Inputs=5
  Wagon model : Subsystem
  Wagon model1 : Subsystem
  Wagon model2 : Subsystem
  Wagon model3 : Subsystem
  Wagon model4 : Subsystem
  Out5 : Outport  VectorParamsAs1DForOutWhenUnconnected=off
  Out17 : Outport  Port=2  VectorParamsAs1DForOutWhenUnconnected=off
  Out2 : Outport  Port=3  VectorParamsAs1DForOutWhenUnconnected=off
  "v_vec " : Outport  Port=4
  wires:
  Wagon model3/2(p_BP_out) -> Mux2/4, Wagon model4/1(p_BP)
  Mux/1 -> Out5/1  "F_vec"
  Wagon model1/2(p_BP_out) -> Mux2/2, Wagon model2/1(p_BP)
  Wagon model4/2(p_BP_out) -> Out17/1, Mux2/5  "p_BP_out"
  Wagon model4/1(Fres) -> Mux/5
  Wagon model2/2(p_BP_out) -> Mux2/3, Wagon model3/1(p_BP)
  Wagon model/2(p_BP_out) -> Mux2/1, Wagon model1/1(p_BP)
  Wagon model3/1(Fres) -> Mux/4
  Wagon model2/1(Fres) -> Mux/3
  Wagon model1/1(Fres) -> Mux/2
  Wagon model/1(Fres) -> Mux/1
  Mux2/1 -> Out2/1  "BP_vec"
  p_BP/1 -> Wagon model/1(p_BP)
  Wagon model/3("v ") -> Mux1/1
  Wagon model1/3("v ") -> Mux1/2
  Wagon model3/3("v ") -> Mux1/3
  Wagon model4/3("v ") -> Mux1/5
  Wagon model2/3("v ") -> Mux1/4
  Mux1/1 -> "v_vec "/1

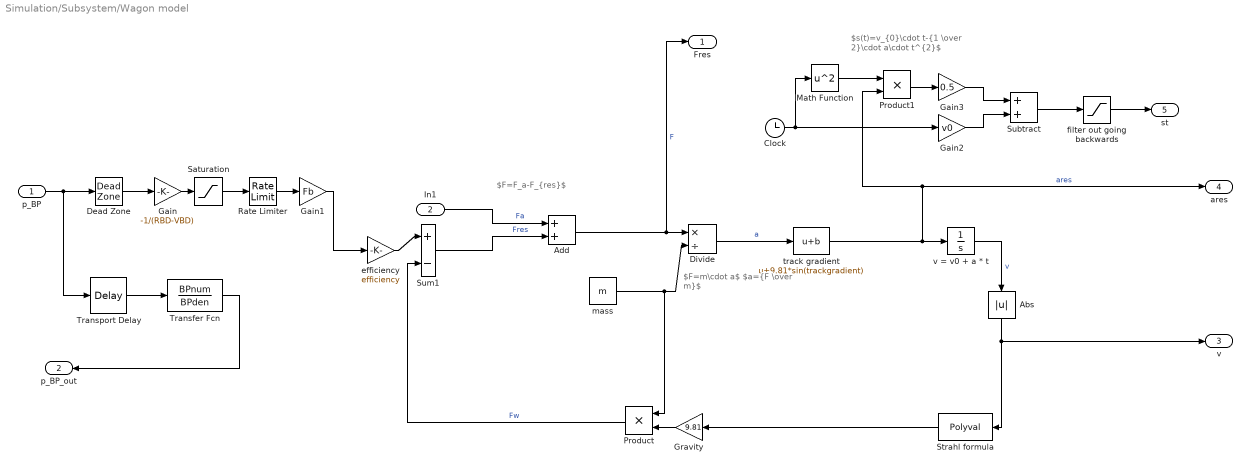
== system Simulation/Subsystem/Wagon model ==
  note: $F=F_a-F_{res}$
  note: $s(t)=v_{0}\cdot t-{1 \over 2}\cdot a\cdot t^{2}$
  note: $F=m\cdot a$ $a={F \over m}$
  p_BP : Inport
  In1 : Inport  Port=2
  Abs : Abs
  Add : Sum
  Clock : Clock
  Dead Zone : DeadZone  LowerValue=-0.001  UpperValue=0.001  SaturateOnIntegerOverflow=on
  Divide : Product  Inputs=*/
  Gain : Gain  Gain=-1/(RBD-VBD)
  Gain1 : Gain  Gain=Fb
  Gain2 : Gain  Gain=v0
  Gain3 : Gain  Gain=0.5
  Gravity : Gain  Gain=9.81
  Math Function : Math  Operator=square  SignedPower=off  SaturateOnIntegerOverflow=on
  Product : Product
  Product1 : Product
  Rate Limiter : RateLimiter  RisingSlewLimit=1/tf  FallingSlewLimit=-1/tl  SampleTimeMode=inherited
  Saturation : Saturate  UpperLimit=1  LowerLimit=0
  Strahl formula : Polyval  Coefs=Pres
  Subtract : Sum
  Sum1 : Sum  Inputs=|+-
  Transfer Fcn : TransferFcn  Numerator=BPnum  Denominator=BPden
  Transport Delay : TransportDelay  DelayTime=l/c  InitialOutput=p0
  efficiency : Gain  Gain=efficiency
  filter out going backwards : Saturate  UpperLimit=inf  LowerLimit=0
  mass : Constant  Value=m
  track gradient : Bias  Bias=9.81*sin(trackgradient)
  v = v0 + a * t : Integrator  InitialCondition=v0
  Fres : Outport  VectorParamsAs1DForOutWhenUnconnected=off
  p_BP_out : Outport  Port=2  VectorParamsAs1DForOutWhenUnconnected=off
  "v " : Outport  Port=3
  ares : Outport  Port=4
  st : Outport  Port=5
  wires:
  Strahl formula/1 -> Gravity/1
  Abs/1 -> "v "/1, Strahl formula/1
  Gravity/1 -> Product/2
  Product/1 -> Sum1/2  "Fw"
  v = v0 + a * t/1 -> Abs/1  "v"
  mass/1 -> Product/1, Divide/2
  Divide/1 -> track gradient/1  "a"
  p_BP/1 -> Transport Delay/1, Dead Zone/1
  Gain/1 -> Saturation/1
  Gain1/1 -> efficiency/1
  Saturation/1 -> Rate Limiter/1
  Rate Limiter/1 -> Gain1/1
  Transfer Fcn/1 -> p_BP_out/1
  Transport Delay/1 -> Transfer Fcn/1
  efficiency/1 -> Sum1/1
  track gradient/1 -> ares/1, Product1/2, v = v0 + a * t/1  "ares"
  Clock/1 -> Math Function/1, Gain2/1
  Math Function/1 -> Product1/1
  Product1/1 -> Gain3/1
  Subtract/1 -> filter out going backwards/1
  Gain3/1 -> Subtract/1
  Gain2/1 -> Subtract/2
  filter out going backwards/1 -> st/1
  Dead Zone/1 -> Gain/1
  In1/1 -> Add/1  "Fa"
  Sum1/1 -> Add/2  "Fres"
  Add/1 -> Fres/1, Divide/1  "F"

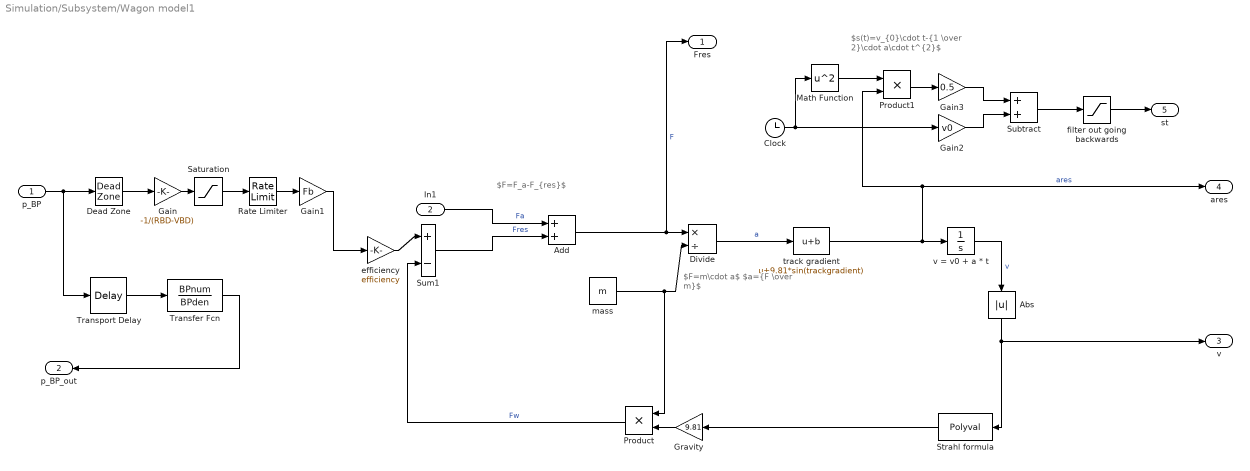
== system Simulation/Subsystem/Wagon model1 ==
  note: $F=F_a-F_{res}$
  note: $s(t)=v_{0}\cdot t-{1 \over 2}\cdot a\cdot t^{2}$
  note: $F=m\cdot a$ $a={F \over m}$
  p_BP : Inport
  In1 : Inport  Port=2
  Abs : Abs
  Add : Sum
  Clock : Clock
  Dead Zone : DeadZone  LowerValue=-0.001  UpperValue=0.001  SaturateOnIntegerOverflow=on
  Divide : Product  Inputs=*/
  Gain : Gain  Gain=-1/(RBD-VBD)
  Gain1 : Gain  Gain=Fb
  Gain2 : Gain  Gain=v0
  Gain3 : Gain  Gain=0.5
  Gravity : Gain  Gain=9.81
  Math Function : Math  Operator=square  SignedPower=off  SaturateOnIntegerOverflow=on
  Product : Product
  Product1 : Product
  Rate Limiter : RateLimiter  RisingSlewLimit=1/tf  FallingSlewLimit=-1/tl  SampleTimeMode=inherited
  Saturation : Saturate  UpperLimit=1  LowerLimit=0
  Strahl formula : Polyval  Coefs=Pres
  Subtract : Sum
  Sum1 : Sum  Inputs=|+-
  Transfer Fcn : TransferFcn  Numerator=BPnum  Denominator=BPden
  Transport Delay : TransportDelay  DelayTime=l/c  InitialOutput=p0
  efficiency : Gain  Gain=efficiency
  filter out going backwards : Saturate  UpperLimit=inf  LowerLimit=0
  mass : Constant  Value=m
  track gradient : Bias  Bias=9.81*sin(trackgradient)
  v = v0 + a * t : Integrator  InitialCondition=v0
  Fres : Outport  VectorParamsAs1DForOutWhenUnconnected=off
  p_BP_out : Outport  Port=2  VectorParamsAs1DForOutWhenUnconnected=off
  "v " : Outport  Port=3
  ares : Outport  Port=4
  st : Outport  Port=5
  wires:
  Strahl formula/1 -> Gravity/1
  Abs/1 -> "v "/1, Strahl formula/1
  Gravity/1 -> Product/2
  Product/1 -> Sum1/2  "Fw"
  v = v0 + a * t/1 -> Abs/1  "v"
  mass/1 -> Product/1, Divide/2
  Divide/1 -> track gradient/1  "a"
  p_BP/1 -> Transport Delay/1, Dead Zone/1
  Gain/1 -> Saturation/1
  Gain1/1 -> efficiency/1
  Saturation/1 -> Rate Limiter/1
  Rate Limiter/1 -> Gain1/1
  Transfer Fcn/1 -> p_BP_out/1
  Transport Delay/1 -> Transfer Fcn/1
  efficiency/1 -> Sum1/1
  track gradient/1 -> ares/1, Product1/2, v = v0 + a * t/1  "ares"
  Clock/1 -> Math Function/1, Gain2/1
  Math Function/1 -> Product1/1
  Product1/1 -> Gain3/1
  Subtract/1 -> filter out going backwards/1
  Gain3/1 -> Subtract/1
  Gain2/1 -> Subtract/2
  filter out going backwards/1 -> st/1
  Dead Zone/1 -> Gain/1
  In1/1 -> Add/1  "Fa"
  Sum1/1 -> Add/2  "Fres"
  Add/1 -> Fres/1, Divide/1  "F"

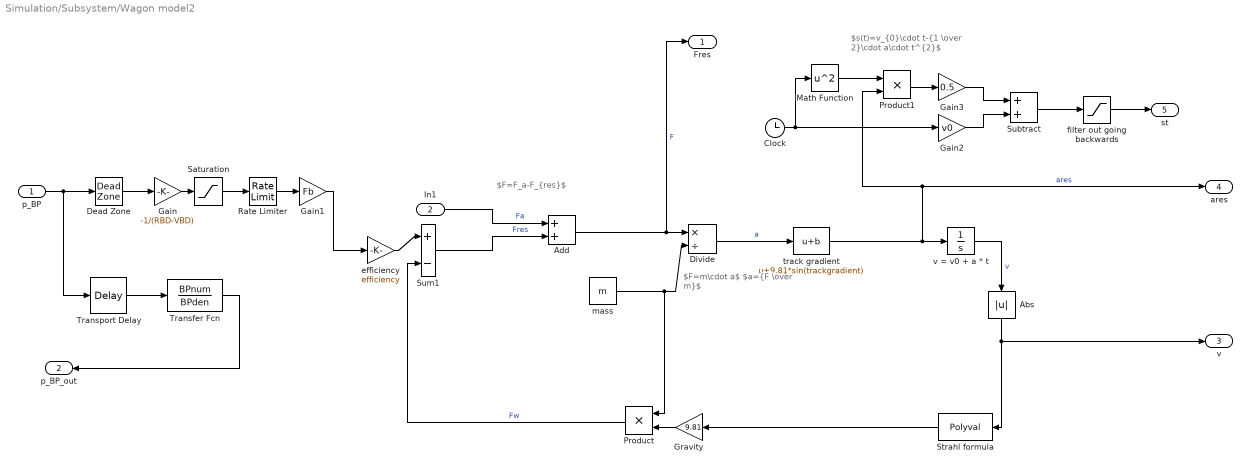
== system Simulation/Subsystem/Wagon model2 ==
  note: $F=F_a-F_{res}$
  note: $s(t)=v_{0}\cdot t-{1 \over 2}\cdot a\cdot t^{2}$
  note: $F=m\cdot a$ $a={F \over m}$
  p_BP : Inport
  In1 : Inport  Port=2
  Abs : Abs
  Add : Sum
  Clock : Clock
  Dead Zone : DeadZone  LowerValue=-0.001  UpperValue=0.001  SaturateOnIntegerOverflow=on
  Divide : Product  Inputs=*/
  Gain : Gain  Gain=-1/(RBD-VBD)
  Gain1 : Gain  Gain=Fb
  Gain2 : Gain  Gain=v0
  Gain3 : Gain  Gain=0.5
  Gravity : Gain  Gain=9.81
  Math Function : Math  Operator=square  SignedPower=off  SaturateOnIntegerOverflow=on
  Product : Product
  Product1 : Product
  Rate Limiter : RateLimiter  RisingSlewLimit=1/tf  FallingSlewLimit=-1/tl  SampleTimeMode=inherited
  Saturation : Saturate  UpperLimit=1  LowerLimit=0
  Strahl formula : Polyval  Coefs=Pres
  Subtract : Sum
  Sum1 : Sum  Inputs=|+-
  Transfer Fcn : TransferFcn  Numerator=BPnum  Denominator=BPden
  Transport Delay : TransportDelay  DelayTime=l/c  InitialOutput=p0
  efficiency : Gain  Gain=efficiency
  filter out going backwards : Saturate  UpperLimit=inf  LowerLimit=0
  mass : Constant  Value=m
  track gradient : Bias  Bias=9.81*sin(trackgradient)
  v = v0 + a * t : Integrator  InitialCondition=v0
  Fres : Outport  VectorParamsAs1DForOutWhenUnconnected=off
  p_BP_out : Outport  Port=2  VectorParamsAs1DForOutWhenUnconnected=off
  "v " : Outport  Port=3
  ares : Outport  Port=4
  st : Outport  Port=5
  wires:
  Strahl formula/1 -> Gravity/1
  Abs/1 -> "v "/1, Strahl formula/1
  Gravity/1 -> Product/2
  Product/1 -> Sum1/2  "Fw"
  v = v0 + a * t/1 -> Abs/1  "v"
  mass/1 -> Product/1, Divide/2
  Divide/1 -> track gradient/1  "a"
  p_BP/1 -> Transport Delay/1, Dead Zone/1
  Gain/1 -> Saturation/1
  Gain1/1 -> efficiency/1
  Saturation/1 -> Rate Limiter/1
  Rate Limiter/1 -> Gain1/1
  Transfer Fcn/1 -> p_BP_out/1
  Transport Delay/1 -> Transfer Fcn/1
  efficiency/1 -> Sum1/1
  track gradient/1 -> ares/1, Product1/2, v = v0 + a * t/1  "ares"
  Clock/1 -> Math Function/1, Gain2/1
  Math Function/1 -> Product1/1
  Product1/1 -> Gain3/1
  Subtract/1 -> filter out going backwards/1
  Gain3/1 -> Subtract/1
  Gain2/1 -> Subtract/2
  filter out going backwards/1 -> st/1
  Dead Zone/1 -> Gain/1
  In1/1 -> Add/1  "Fa"
  Sum1/1 -> Add/2  "Fres"
  Add/1 -> Fres/1, Divide/1  "F"

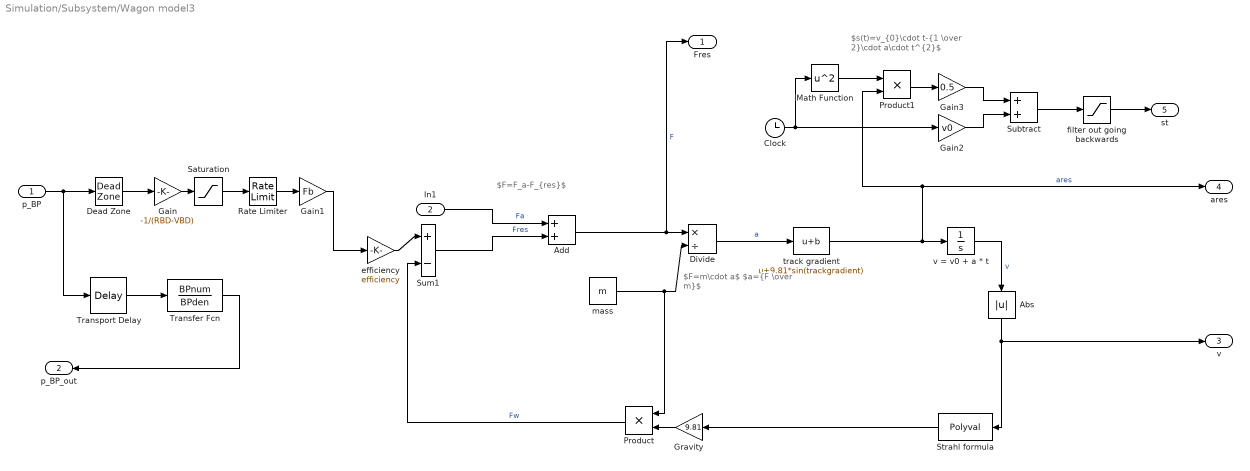
== system Simulation/Subsystem/Wagon model3 ==
  note: $F=F_a-F_{res}$
  note: $s(t)=v_{0}\cdot t-{1 \over 2}\cdot a\cdot t^{2}$
  note: $F=m\cdot a$ $a={F \over m}$
  p_BP : Inport
  In1 : Inport  Port=2
  Abs : Abs
  Add : Sum
  Clock : Clock
  Dead Zone : DeadZone  LowerValue=-0.001  UpperValue=0.001  SaturateOnIntegerOverflow=on
  Divide : Product  Inputs=*/
  Gain : Gain  Gain=-1/(RBD-VBD)
  Gain1 : Gain  Gain=Fb
  Gain2 : Gain  Gain=v0
  Gain3 : Gain  Gain=0.5
  Gravity : Gain  Gain=9.81
  Math Function : Math  Operator=square  SignedPower=off  SaturateOnIntegerOverflow=on
  Product : Product
  Product1 : Product
  Rate Limiter : RateLimiter  RisingSlewLimit=1/tf  FallingSlewLimit=-1/tl  SampleTimeMode=inherited
  Saturation : Saturate  UpperLimit=1  LowerLimit=0
  Strahl formula : Polyval  Coefs=Pres
  Subtract : Sum
  Sum1 : Sum  Inputs=|+-
  Transfer Fcn : TransferFcn  Numerator=BPnum  Denominator=BPden
  Transport Delay : TransportDelay  DelayTime=l/c  InitialOutput=p0
  efficiency : Gain  Gain=efficiency
  filter out going backwards : Saturate  UpperLimit=inf  LowerLimit=0
  mass : Constant  Value=m
  track gradient : Bias  Bias=9.81*sin(trackgradient)
  v = v0 + a * t : Integrator  InitialCondition=v0
  Fres : Outport  VectorParamsAs1DForOutWhenUnconnected=off
  p_BP_out : Outport  Port=2  VectorParamsAs1DForOutWhenUnconnected=off
  "v " : Outport  Port=3
  ares : Outport  Port=4
  st : Outport  Port=5
  wires:
  Strahl formula/1 -> Gravity/1
  Abs/1 -> "v "/1, Strahl formula/1
  Gravity/1 -> Product/2
  Product/1 -> Sum1/2  "Fw"
  v = v0 + a * t/1 -> Abs/1  "v"
  mass/1 -> Product/1, Divide/2
  Divide/1 -> track gradient/1  "a"
  p_BP/1 -> Transport Delay/1, Dead Zone/1
  Gain/1 -> Saturation/1
  Gain1/1 -> efficiency/1
  Saturation/1 -> Rate Limiter/1
  Rate Limiter/1 -> Gain1/1
  Transfer Fcn/1 -> p_BP_out/1
  Transport Delay/1 -> Transfer Fcn/1
  efficiency/1 -> Sum1/1
  track gradient/1 -> ares/1, Product1/2, v = v0 + a * t/1  "ares"
  Clock/1 -> Math Function/1, Gain2/1
  Math Function/1 -> Product1/1
  Product1/1 -> Gain3/1
  Subtract/1 -> filter out going backwards/1
  Gain3/1 -> Subtract/1
  Gain2/1 -> Subtract/2
  filter out going backwards/1 -> st/1
  Dead Zone/1 -> Gain/1
  In1/1 -> Add/1  "Fa"
  Sum1/1 -> Add/2  "Fres"
  Add/1 -> Fres/1, Divide/1  "F"

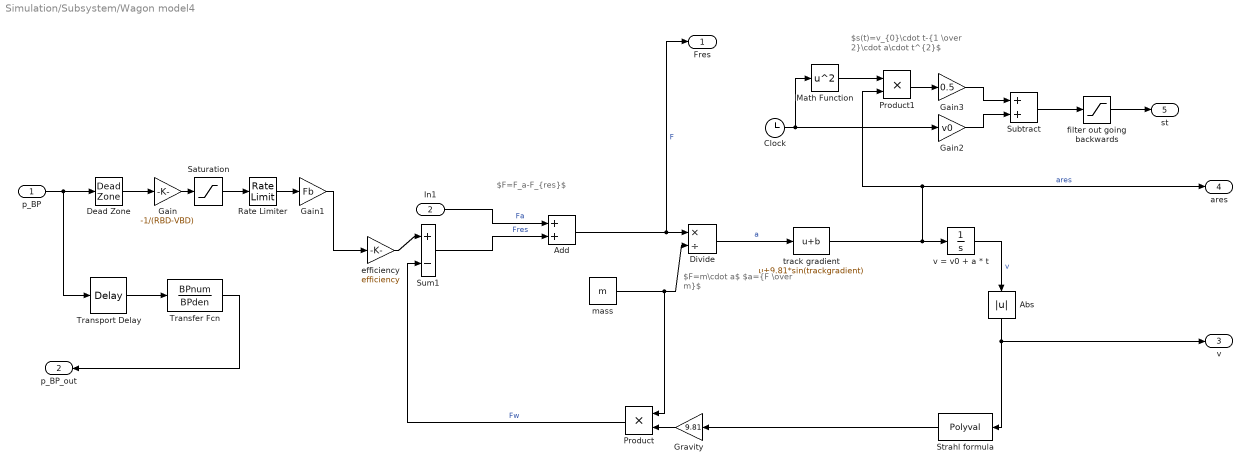
== system Simulation/Subsystem/Wagon model4 ==
  note: $F=F_a-F_{res}$
  note: $s(t)=v_{0}\cdot t-{1 \over 2}\cdot a\cdot t^{2}$
  note: $F=m\cdot a$ $a={F \over m}$
  p_BP : Inport
  In1 : Inport  Port=2
  Abs : Abs
  Add : Sum
  Clock : Clock
  Dead Zone : DeadZone  LowerValue=-0.001  UpperValue=0.001  SaturateOnIntegerOverflow=on
  Divide : Product  Inputs=*/
  Gain : Gain  Gain=-1/(RBD-VBD)
  Gain1 : Gain  Gain=Fb
  Gain2 : Gain  Gain=v0
  Gain3 : Gain  Gain=0.5
  Gravity : Gain  Gain=9.81
  Math Function : Math  Operator=square  SignedPower=off  SaturateOnIntegerOverflow=on
  Product : Product
  Product1 : Product
  Rate Limiter : RateLimiter  RisingSlewLimit=1/tf  FallingSlewLimit=-1/tl  SampleTimeMode=inherited
  Saturation : Saturate  UpperLimit=1  LowerLimit=0
  Strahl formula : Polyval  Coefs=Pres
  Subtract : Sum
  Sum1 : Sum  Inputs=|+-
  Transfer Fcn : TransferFcn  Numerator=BPnum  Denominator=BPden
  Transport Delay : TransportDelay  DelayTime=l/c  InitialOutput=p0
  efficiency : Gain  Gain=efficiency
  filter out going backwards : Saturate  UpperLimit=inf  LowerLimit=0
  mass : Constant  Value=m
  track gradient : Bias  Bias=9.81*sin(trackgradient)
  v = v0 + a * t : Integrator  InitialCondition=v0
  Fres : Outport  VectorParamsAs1DForOutWhenUnconnected=off
  p_BP_out : Outport  Port=2  VectorParamsAs1DForOutWhenUnconnected=off
  "v " : Outport  Port=3
  ares : Outport  Port=4
  st : Outport  Port=5
  wires:
  Strahl formula/1 -> Gravity/1
  Abs/1 -> "v "/1, Strahl formula/1
  Gravity/1 -> Product/2
  Product/1 -> Sum1/2  "Fw"
  v = v0 + a * t/1 -> Abs/1  "v"
  mass/1 -> Product/1, Divide/2
  Divide/1 -> track gradient/1  "a"
  p_BP/1 -> Transport Delay/1, Dead Zone/1
  Gain/1 -> Saturation/1
  Gain1/1 -> efficiency/1
  Saturation/1 -> Rate Limiter/1
  Rate Limiter/1 -> Gain1/1
  Transfer Fcn/1 -> p_BP_out/1
  Transport Delay/1 -> Transfer Fcn/1
  efficiency/1 -> Sum1/1
  track gradient/1 -> ares/1, Product1/2, v = v0 + a * t/1  "ares"
  Clock/1 -> Math Function/1, Gain2/1
  Math Function/1 -> Product1/1
  Product1/1 -> Gain3/1
  Subtract/1 -> filter out going backwards/1
  Gain3/1 -> Subtract/1
  Gain2/1 -> Subtract/2
  filter out going backwards/1 -> st/1
  Dead Zone/1 -> Gain/1
  In1/1 -> Add/1  "Fa"
  Sum1/1 -> Add/2  "Fres"
  Add/1 -> Fres/1, Divide/1  "F"

== system Simulation/Subsystem1/Wagon model ==
  note: $F=F_a-F_{res}$
  note: $s(t)=v_{0}\cdot t-{1 \over 2}\cdot a\cdot t^{2}$
  note: $F=m\cdot a$ $a={F \over m}$
  p_BP : Inport
  In1 : Inport  Port=2
  Abs : Abs
  Add : Sum
  Clock : Clock
  Dead Zone : DeadZone  LowerValue=-0.001  UpperValue=0.001  SaturateOnIntegerOverflow=on
  Divide : Product  Inputs=*/
  Gain : Gain  Gain=-1/(RBD-VBD)
  Gain1 : Gain  Gain=Fb
  Gain2 : Gain  Gain=v0
  Gain3 : Gain  Gain=0.5
  Gravity : Gain  Gain=9.81
  Math Function : Math  Operator=square  SignedPower=off  SaturateOnIntegerOverflow=on
  Product : Product
  Product1 : Product
  Rate Limiter : RateLimiter  RisingSlewLimit=1/tf  FallingSlewLimit=-1/tl  SampleTimeMode=inherited
  Saturation : Saturate  UpperLimit=1  LowerLimit=0
  Strahl formula : Polyval  Coefs=Pres
  Subtract : Sum
  Sum1 : Sum  Inputs=|+-
  Transfer Fcn : TransferFcn  Numerator=BPnum  Denominator=BPden
  Transport Delay : TransportDelay  DelayTime=l/c  InitialOutput=p0
  efficiency : Gain  Gain=efficiency
  filter out going backwards : Saturate  UpperLimit=inf  LowerLimit=0
  mass : Constant  Value=m
  track gradient : Bias  Bias=9.81*sin(trackgradient)
  v = v0 + a * t : Integrator  InitialCondition=v0
  Fres : Outport  VectorParamsAs1DForOutWhenUnconnected=off
  p_BP_out : Outport  Port=2  VectorParamsAs1DForOutWhenUnconnected=off
  "v " : Outport  Port=3
  ares : Outport  Port=4
  st : Outport  Port=5
  wires:
  Strahl formula/1 -> Gravity/1
  Abs/1 -> "v "/1, Strahl formula/1
  Gravity/1 -> Product/2
  Product/1 -> Sum1/2  "Fw"
  v = v0 + a * t/1 -> Abs/1  "v"
  mass/1 -> Product/1, Divide/2
  Divide/1 -> track gradient/1  "a"
  p_BP/1 -> Transport Delay/1, Dead Zone/1
  Gain/1 -> Saturation/1
  Gain1/1 -> efficiency/1
  Saturation/1 -> Rate Limiter/1
  Rate Limiter/1 -> Gain1/1
  Transfer Fcn/1 -> p_BP_out/1
  Transport Delay/1 -> Transfer Fcn/1
  efficiency/1 -> Sum1/1
  track gradient/1 -> ares/1, Product1/2, v = v0 + a * t/1  "ares"
  Clock/1 -> Math Function/1, Gain2/1
  Math Function/1 -> Product1/1
  Product1/1 -> Gain3/1
  Subtract/1 -> filter out going backwards/1
  Gain3/1 -> Subtract/1
  Gain2/1 -> Subtract/2
  filter out going backwards/1 -> st/1
  Dead Zone/1 -> Gain/1
  In1/1 -> Add/1  "Fa"
  Sum1/1 -> Add/2  "Fres"
  Add/1 -> Fres/1, Divide/1  "F"
